simulink model "paper_Exponential_Predefined_102"  (R2019a)
settings: Solver=ode4  StartTime=0.0  StopTime=40  FixedStep=0.001  RelTol=1e-3
libraries: simulink x6
(part 3 of 3)

== matlab function paper_Exponential_Predefined_102/control input 5 ==
  data: a_xr input; a_yr input; a_zr input; psi input; gamma input; u1_omiga_psi output; u2_omiga_gamma output; u3_a output; v input; nta_1 input; nta_2 input; nta_3 input
function [u1_omiga_psi,u2_omiga_gamma,u3_a] = fcn(a_xr,a_yr,a_zr,psi,gamma,v,nta_1,nta_2,nta_3)
A = [-a_xr;-a_yr;-a_zr];
B = [-v*sin(psi)*cos(gamma) -v*cos(psi)*sin(gamma) cos(psi)*cos(gamma); 
    v*cos(psi)*cos(gamma) -v*sin(psi)*sin(gamma) sin(psi)*cos(gamma);
    0                        v*cos(gamma)               sin(gamma)];
nta = [nta_1 ; nta_2;nta_3];
U = -inv(B)*(A - nta);
U11=U(1,1); 
U21=U(2,1);
U31=U(3,1);
% 

u1_omiga_psi = U11 ;
u2_omiga_gamma = U21;
u3_a =U31 ;
%%添加约束





end

== matlab function paper_Exponential_Predefined_102/f,df5 ==
  data: dx input; x input; dy input; y input; dz input; z input; dxr input; xr input; dyr input; yr input; dzr input; zr input; p1x output; p1y output; p1z output; p2x output; p2y output; p2z output; wx input; wy input; wz input; s1 output; s2 output; s3 output
 function [p1x,p1y,p1z,p2x,p2y,p2z,s1,s2,s3] = fcn(dx,x,dy,y,dz,z,dxr,xr,dyr,yr,dzr,zr,wx,wy,wz)
% wx=0;
% wy=0;
% wz=0;
p1x = x - xr;
p1y = y - yr;
p1z = z - zr;
s1 = dx - dxr ;
s2 = dy - dyr ;
s3 = dz - dzr ;
p2x = dx - dxr-wx ;
p2y = dy - dyr-wy ;
p2z = dz - dzr-wz ;
end

== matlab function paper_Exponential_Predefined_102/u_1a5 ==
  data: u input; u_1a output
 function u_1a  = fcn(u)

u_max=1.6;

u_1a=u_max*erf((pi^(0.5)*u)/(2*u_max));


 end

== matlab function paper_Exponential_Predefined_102/u_2a6 ==
  data: u input; u_2a output
function u_2a  = fcn(u)

u_max=1.6;

u_2a=u_max*erf((pi^(0.5)*u)/(2*u_max));


 end

== matlab function paper_Exponential_Predefined_102/u_3a5 ==
  data: u input; u_3a output
function u_3a  = fcn(u)

u_max=17;

u_3a=u_max*erf((pi^(0.5)*u)/(2*u_max));

 end

== matlab function paper_Exponential_Predefined_102/yuding_zhishu5 ==
  data: t input; nta_1 output; t_f input; bta1 input; bta2 input; k1 input; k2 input; p1x input; p1y input; p1z input; p2x input; p2y input; p2z input; z2x input; z2y input; z2z input; nta_2 output; nta_3 output
function [nta_1,nta_2,nta_3] = yuding(t,t_f,bta1,bta2,k1,k2,p1x,p1y,p1z,p2x,p2y,p2z,z2x,z2y,z2z)

x2d=-k1*p1x;
y2d=-k1*p1y;
z2d=-k1*p1z;
sigama2x=p2x-x2d;
sigama2y=p2y-y2d;
sigama2z=p2z-z2d;

nta_1=-p1x+k1-k2*sigama2x-z2x;

nta_2=-p1y+k1-k2*sigama2y-z2y;

nta_3=-p1z+k1-k2*sigama2z-z2z;

   
end

== matlab function paper_Exponential_Predefined_102/ref_UAV ==
  data: ar input; vr input; a_xr output; a_yr output; omiga_psi_r input; psi_r input; omiga_gamma_r input; a_zr output; gamma_r input
function [a_xr,a_yr,a_zr] = fcn(ar,vr,omiga_psi_r,psi_r,omiga_gamma_r,gamma_r)
%a_r=\ddot x^r 
a_xr = -vr*sin(psi_r)*cos(gamma_r)*omiga_psi_r-vr*cos(psi_r)*sin(gamma_r)*omiga_gamma_r+cos(psi_r)*cos(gamma_r)*ar;
a_yr = vr*cos(psi_r)*cos(gamma_r)*omiga_psi_r-vr*sin(psi_r)*sin(gamma_r)*omiga_gamma_r+ sin(psi_r)*cos(gamma_r)*ar;
a_zr = vr*cos(gamma_r)*omiga_gamma_r + sin(gamma_r)*ar;
end

== matlab function paper_Exponential_Predefined_102/MATLAB Function21 ==
  data: p1y input; p2y input; z0y input; dz0y output; dz1y output; dz2y output; z1y input; z2y input
function [dz0y,dz1y,dz2y] = FTDO(p1y,p2y,z0y,z1y,z2y)
r=[24 216 864];%parameters of FTDO
r0=r(1);
r1=r(2);
r2=r(3);
v0=-r0*(abs(z0y-p1y))^(0.8)*sign(z0y-p1y)-r0*(abs(z0y-p1y))^(1.2)*sign(z0y-p1y)+z1y;
dz0y=v0+p2y;
v1=-r1*(abs(z0y-p1y))^(0.6)*sign(z0y-p1y)-r1*(abs(z0y-p1y))^(1.4)*sign(z0y-p1y)+z2y;
dz1y=v1;
dz2y =-r2*(abs(z0y-p1y))^(0.4)*sign(z0y-p1y)-r2*(abs(z0y-p1y))^(1.6)*sign(z0y-p1y);
end

== matlab function paper_Exponential_Predefined_102/MATLAB Function22 ==
  data: t input; dx output; dy output; dz output; delta input; v input; gamma input; psi input
function [dx,dy,dz] = disturbance(t,delta,v,gamma,psi)
% w is the wind disturbance and h is the unmodelled dynamics of the UAV 
% The parameter setting is the same as the simulation part B. Case 2 in the paper

hx=-0.0005*abs(v-36)*exp((0.4*v)^0.5)+0.2*sin(psi);
hy=-0.0004*abs(v-30)*exp((0.3*v)^0.5)+0.2*cos(psi);
hz=-0.004*v^(0.5)*sin(3*gamma);

if 0<t && t<10
    wx = 1*sin(t)+delta;
else
    wx=0;
end
if 5<t && t<15
    wy = 2*sin(2*t)-cos(3*t)+delta;
else
    wy=0;
end
if 0<t && t<20
    wz = 0.5*sin(t)+delta;
else
    wz = 0;
end

dx=hx+wx;
dy=hy+wy;
dz=hz+wz;

end

== matlab function paper_Exponential_Predefined_102/MATLAB Function23 ==
  data: p1z input; p2z input; z0z input; dz0z output; dz1z output; dz2z output; z1z input; z2z input
function [dz0z,dz1z,dz2z] = FTDO(p1z,p2z,z0z,z1z,z2z)
r=[24 216 864];%parameters of FTDO
r0=r(1);
r1=r(2);
r2=r(3);
v0=-r0*(abs(z0z-p1z))^(0.8)*sign(z0z-p1z)-r0*(abs(z0z-p1z))^(1.2)*sign(z0z-p1z)+z1z;
dz0z=v0+p2z;
v1=-r1*(abs(z0z-p1z))^(0.6)*sign(z0z-p1z)-r1*(abs(z0z-p1z))^(1.4)*sign(z0z-p1z)+z2z;
dz1z=v1;
dz2z =-r2*(abs(z0z-p1z))^(0.4)*sign(z0z-p1z)-r2*(abs(z0z-p1z))^(1.6)*sign(z0z-p1z);
end

== matlab function paper_Exponential_Predefined_102/MATLAB Function24 ==
  data: p1x input; p2x input; z0x input; dz0x output; dz1x output; dz2x output; z1x input; z2x input
function [dz0x,dz1x,dz2x] = FTDO(p1x,p2x,z0x,z1x,z2x)
r=[24 216 864];%parameters of FTDO
r0=r(1);
r1=r(2);
r2=r(3);
v0=-r0*(abs(z0x-p1x))^(0.8)*sign(z0x-p1x)-r0*(abs(z0x-p1x))^(1.2)*sign(z0x-p1x)+z1x;
dz0x=v0+p2x;
v1=-r1*(abs(z0x-p1x))^(0.6)*sign(z0x-p1x)-r1*(abs(z0x-p1x))^(1.4)*sign(z0x-p1x)+z2x;
dz1x=v1;
dz2x =-r2*(abs(z0x-p1x))^(0.4)*sign(z0x-p1x)-r2*(abs(z0x-p1x))^(1.6)*sign(z0x-p1x);
end

== matlab function paper_Exponential_Predefined_102/X_dot6 ==
  data: vr input; psi_r input; gamma_r input; psi input; gamma input; v input; dx output; dy output; dz output; xr_dot output; yr_dot output; zr_dot output; wx input; wy input; wz input
function [dx,dy,dz,xr_dot,yr_dot,zr_dot] = dot_state(vr,psi_r,gamma_r,psi,gamma,v,wx,wy,wz)
%dx,dy,dz is the derivative of position. wx,wy,wz is the wind disturbances
dx = v*cos(psi)*cos(gamma)+wx; 
dy = v*sin(psi)*cos(gamma)+wy;
dz = v*sin(gamma)+wz;
xr_dot = vr*cos(psi_r)*cos(gamma_r);
yr_dot = vr*sin(psi_r)*cos(gamma_r);
zr_dot = vr*sin(gamma_r);
end

== matlab function paper_Exponential_Predefined_102/U ==
  data: a_xr input; a_yr input; a_zr input; psi input; gamma input; u1_omiga_psi output; u2_omiga_gamma output; u3_a output; v input; qnta_1 input; qnta_2 input; qnta_3 input
function [u1_omiga_psi,u2_omiga_gamma,u3_a] = fcn(a_xr,a_yr,a_zr,psi,gamma,v,qnta_1,qnta_2,qnta_3)
%A,B,U,qnta corresponds to the matrix of formula (40) in the paper
A = [-a_xr;-a_yr;-a_zr];
B = [-v*sin(psi)*cos(gamma) -v*cos(psi)*sin(gamma) cos(psi)*cos(gamma); 
    v*cos(psi)*cos(gamma) -v*sin(psi)*sin(gamma) sin(psi)*cos(gamma);
    0                        v*cos(gamma)               sin(gamma)];
qnta = [qnta_1 ; qnta_2;qnta_3];
U = -inv(B)*( - qnta);
U11=U(1,1); 
U21=U(2,1);
U31=U(3,1);


u1_omiga_psi = U11 ;
u2_omiga_gamma = U21;
u3_a =U31 ;






end

== matlab function paper_Exponential_Predefined_102/sys ==
  data: dx input; x input; dy input; y input; dz input; z input; dxr input; xr input; dyr input; yr input; dzr input; zr input; p1x output; p1y output; p1z output; p2x output; p2y output; p2z output; wx input; wy input; wz input; s1 output; s2 output; s3 output
 function [p1x,p1y,p1z,p2x,p2y,p2z,s1,s2,s3] = sys(dx,x,dy,y,dz,z,dxr,xr,dyr,yr,dzr,zr,wx,wy,wz)
%p1,p2,s corresponds to the matrix of formula (53) in the paper
p1x = x - xr;
p1y = y - yr;
p1z = z - zr;
s1 = dx - dxr ;
s2 = dy - dyr ;
s3 = dz - dzr ;
p2x = dx - dxr-wx ;
p2y = dy - dyr-wy ;
p2z = dz - dzr-wz ;
end

== matlab function paper_Exponential_Predefined_102/qnta ==
  data: nta1 input; qnta1 output; nta2 input; nta3 input; qnta2 output; qnta3 output
function [qnta1,qnta2,qnta3]= qnta(nta1,nta2,nta3)
%% qnta corresponds to the matrix of formula (51) in the paper
nta_1max=10;
nta_2max=10;
nta_3max=10;
% nta_1max=15;
% nta_2max=15;
% nta_3max=15;
qnta1=nta_1max*erf((pi^(0.5)*nta1)/(2*nta_1max));
qnta2=nta_2max*erf((pi^(0.5)*nta2)/(2*nta_2max));
qnta3=nta_3max*erf((pi^(0.5)*nta3)/(2*nta_3max));

 end

== matlab function paper_Exponential_Predefined_102/predefined ==
  data: t input; nta_1 output; t_f input; bta1 input; bta2 input; k1 input; k2 input; p1x input; p1y input; p1z input; p2x input; p2y input; p2z input; z2x input; z2y input; z2z input; nta_2 output; nta_3 output; tua1 input; tua2 input; tua3 input; a_xr input; a_yr input; a_zr input
function [nta_1,nta_2,nta_3] = ex_predefined(t,t_f,bta1,bta2,k1,k2,p1x,p1y,p1z,p2x,p2y,p2z,z2x,z2y,z2z,tua1,tua2,tua3,a_xr,a_yr,a_zr)
%% nta_i corresponds to the matrix of formula (60) in the paper


if  t<t_f
[nta_1,nta_2,nta_3]=Exponential_predefined_sat(t,t_f,bta1,bta2,k1,k2,p1x,p1y,p1z,p2x,p2y,p2z,z2x,z2y,z2z,tua1,tua2,tua3);
else 

    tf=t_f;
    deta_tf=20;    %The control law is cycled every 20 seconds

    if tf<=t & t<(tf+deta_tf)
        [nta_1,nta_2,nta_3]=Exponential_predefined_sat(t,tf+deta_tf,bta1,bta2,k1,k2,p1x,p1y,p1z,p2x,p2y,p2z,z2x,z2y,z2z,tua1,tua2,tua3); 
    else 
        tf=tf+deta_tf;
        [nta_1,nta_2,nta_3]=Exponential_predefined_sat(t,tf+deta_tf,bta1,bta2,k1,k2,p1x,p1y,p1z,p2x,p2y,p2z,z2x,z2y,z2z,tua1,tua2,tua3); 
    end   
    if tf<=t & t<(tf+deta_tf)
        [nta_1,nta_2,nta_3]=Exponential_predefined_sat(t,tf+deta_tf,bta1,bta2,k1,k2,p1x,p1y,p1z,p2x,p2y,p2z,z2x,z2y,z2z,tua1,tua2,tua3); 
    else
        tf=tf+deta_tf;
        [nta_1,nta_2,nta_3]=Exponential_predefined_sat(t,tf+deta_tf,bta1,bta2,k1,k2,p1x,p1y,p1z,p2x,p2y,p2z,z2x,z2y,z2z,tua1,tua2,tua3); 
    end  
    if tf<=t & t<(tf+deta_tf)
        [nta_1,nta_2,nta_3]=Exponential_predefined_sat(t,tf+deta_tf,bta1,bta2,k1,k2,p1x,p1y,p1z,p2x,p2y,p2z,z2x,z2y,z2z,tua1,tua2,tua3); 
    else
        tf=tf+deta_tf;
        [nta_1,nta_2,nta_3]=Exponential_predefined_sat(t,tf+deta_tf,bta1,bta2,k1,k2,p1x,p1y,p1z,p2x,p2y,p2z,z2x,z2y,z2z,tua1,tua2,tua3); 
    end  

    if tf<=t & t<(tf+deta_tf)
        [nta_1,nta_2,nta_3]=Exponential_predefined_sat(t,tf+deta_tf,bta1,bta2,k1,k2,p1x,p1y,p1z,p2x,p2y,p2z,z2x,z2y,z2z,tua1,tua2,tua3); 
    else
        tf=tf+deta_tf;
        [nta_1,nta_2,nta_3]=Exponential_predefined_sat(t,tf+deta_tf,bta1,bta2,k1,k2,p1x,p1y,p1z,p2x,p2y,p2z,z2x,z2y,z2z,tua1,tua2,tua3); 
    end  
end
A = [-a_xr;-a_yr;-a_zr];
nta_1=nta_1-A(1);
nta_2=nta_2-A(2);
nta_3=nta_3-A(3); 
end
